simulink model "PVArray_MPPT"  (R2020b)
settings: Solver=VariableStepAuto  StartTime=0.0  StopTime=1  FixedStep=Ts_Power  RelTol=0.001
PreLoadFcn:
  | Ts_Power=5e-4;
  | Slope_Vdc=1;
InitFcn:
  | Ts_Power=50e-6;
  | Tc=1e-5;%break algebraic loop time constant
StopFcn:
  | if exist('I','var') && exist('V','var')
  |    figure(1)
  |    clf
  |    n=find(I>=0);
  |    n=n(end);
  |    Vglobal=V(1:n);
  |    Iglobal=I(1:n);
  | 
  | 
  |    Pglobal=Vglobal.*Iglobal;
  |    n=find(Pglobal==max(Pglobal));
  |    Pmax=Pglobal(n);
  |    Vmp=Vglobal(n);
  |    Imp=Iglobal(n);
  | 
  | 
  |    subplot(211)
  |    plot(Vglobal, Iglobal,Vmp,Imp,'or')
  |    ylabel('Current (A)')
  |    title(sprintf('Global I-V & P-V characteristics\n %s' ,ModuleName))
  | 
  | 
  |    subplot(212)
  |    plot(Vglobal, Pglobal,Vmp,Pmax,'or')
  |    ylabel('Power (W)')
  |    xlabel('Voltage (V)')
  | end
model workspace (MAT data in the model file):
  slope_Vdc = 3.0848387096
libraries: powerlib x60, re_lib x28, simulink x1
(part 2 of 2)

== system PVArray_MPPT/PV2 ==
  Gate : Inport
  Irr : Inport  Port=2
  1PΩ : Constant  Value=1e15
  Ideal Switch : powerlib/Power Electronics/Ideal Switch  Ron=1e-15  Lon=0  IC=0  Rs=1e15  Cs=inf  Measurements=on
  PV1 : re_lib/Solar/PV Array  Npar=1  Nser=1  PlotType=array @ 25 deg.C & specified irradiances  S_vec="[ 1000  500  100 ]"  Temp_C_vec="[ 45 25  ]"  ModuleName=User-defined  PlotWhenSelected=off  Pm=3.9326  Ncell=1  Voc=0.7712096774  Isc=6.18  Vm=0.6676774194  Im=5.89  beta_Voc_pc=-0.2256195755  alpha_Isc_pc=0.04692556634  beta_Voc=-0.00174  alpha_Isc=0.0029  IL=6.2063  I0=6.3357e-13  nI=1.0041  Rsh=6.9252  Rs=0.0032344  RobustModel=on  RobustCellTemperature=25  BAL=on  Tc=1e-5  Tfilter=5e-5
  Terminator : Terminator
  Terminator1 : Terminator
  Variable Resistor2 : powerlib/Elements/Variable Resistor  Rabsmin=1e-3
      settings: SourceProductBaseCode=PS
  + : PMIOPort  Side=Left
  SW : PMIOPort  Port=2  Side=Right
  - : PMIOPort  Port=3  Side=Right
  wires:
  Gate/1 -> Ideal Switch/1
  Irr/1 -> PV1/1
  1PΩ/1 -> Variable Resistor2/1
  Ideal Switch/1 -> Terminator/1
  PV1/1 -> Terminator1/1
  connections:
  Ideal Switch/RConn1 -- SW/RConn1
  Variable Resistor2/RConn1 -- PV1/RConn2 -- -/RConn1
  +/RConn1 -- Variable Resistor2/LConn1 -- Ideal Switch/LConn1 -- PV1/RConn1

== system PVArray_MPPT/PV20 ==
  Gate : Inport
  Irr : Inport  Port=2
  1PΩ : Constant  Value=1e15
  Ideal Switch : powerlib/Power Electronics/Ideal Switch  Ron=1e-15  Lon=0  IC=0  Rs=1e15  Cs=inf  Measurements=on
  PV1 : re_lib/Solar/PV Array  Npar=1  Nser=1  PlotType=array @ 25 deg.C & specified irradiances  S_vec="[ 1000  500  100 ]"  Temp_C_vec="[ 45 25  ]"  ModuleName=User-defined  PlotWhenSelected=off  Pm=3.9326  Ncell=1  Voc=0.7712096774  Isc=6.18  Vm=0.6676774194  Im=5.89  beta_Voc_pc=-0.2256195755  alpha_Isc_pc=0.04692556634  beta_Voc=-0.00174  alpha_Isc=0.0029  IL=6.2063  I0=6.3357e-13  nI=1.0041  Rsh=6.9252  Rs=0.0032344  RobustModel=on  RobustCellTemperature=25  BAL=on  Tc=1e-5  Tfilter=5e-5
  Terminator : Terminator
  Terminator1 : Terminator
  Variable Resistor2 : powerlib/Elements/Variable Resistor  Rabsmin=1e-3
      settings: SourceProductBaseCode=PS
  + : PMIOPort  Side=Left
  SW : PMIOPort  Port=2  Side=Right
  - : PMIOPort  Port=3  Side=Right
  wires:
  Gate/1 -> Ideal Switch/1
  Irr/1 -> PV1/1
  1PΩ/1 -> Variable Resistor2/1
  Ideal Switch/1 -> Terminator/1
  PV1/1 -> Terminator1/1
  connections:
  Ideal Switch/RConn1 -- SW/RConn1
  Variable Resistor2/RConn1 -- PV1/RConn2 -- -/RConn1
  +/RConn1 -- Variable Resistor2/LConn1 -- Ideal Switch/LConn1 -- PV1/RConn1

== system PVArray_MPPT/PV21 ==
  Gate : Inport
  Irr : Inport  Port=2
  1PΩ : Constant  Value=1e15
  Ideal Switch : powerlib/Power Electronics/Ideal Switch  Ron=1e-15  Lon=0  IC=0  Rs=1e15  Cs=inf  Measurements=on
  PV1 : re_lib/Solar/PV Array  Npar=1  Nser=1  PlotType=array @ 25 deg.C & specified irradiances  S_vec="[ 1000  500  100 ]"  Temp_C_vec="[ 45 25  ]"  ModuleName=User-defined  PlotWhenSelected=off  Pm=3.9326  Ncell=1  Voc=0.7712096774  Isc=6.18  Vm=0.6676774194  Im=5.89  beta_Voc_pc=-0.2256195755  alpha_Isc_pc=0.04692556634  beta_Voc=-0.00174  alpha_Isc=0.0029  IL=6.2063  I0=6.3357e-13  nI=1.0041  Rsh=6.9252  Rs=0.0032344  RobustModel=on  RobustCellTemperature=25  BAL=on  Tc=1e-5  Tfilter=5e-5
  Terminator : Terminator
  Terminator1 : Terminator
  Variable Resistor2 : powerlib/Elements/Variable Resistor  Rabsmin=1e-3
      settings: SourceProductBaseCode=PS
  + : PMIOPort  Side=Left
  SW : PMIOPort  Port=2  Side=Right
  - : PMIOPort  Port=3  Side=Right
  wires:
  Gate/1 -> Ideal Switch/1
  Irr/1 -> PV1/1
  1PΩ/1 -> Variable Resistor2/1
  Ideal Switch/1 -> Terminator/1
  PV1/1 -> Terminator1/1
  connections:
  Ideal Switch/RConn1 -- SW/RConn1
  Variable Resistor2/RConn1 -- PV1/RConn2 -- -/RConn1
  +/RConn1 -- Variable Resistor2/LConn1 -- Ideal Switch/LConn1 -- PV1/RConn1

== system PVArray_MPPT/PV22 ==
  Gate : Inport
  Irr : Inport  Port=2
  1PΩ : Constant  Value=1e15
  Ideal Switch : powerlib/Power Electronics/Ideal Switch  Ron=1e-15  Lon=0  IC=0  Rs=1e15  Cs=inf  Measurements=on
  PV1 : re_lib/Solar/PV Array  Npar=1  Nser=1  PlotType=array @ 25 deg.C & specified irradiances  S_vec="[ 1000  500  100 ]"  Temp_C_vec="[ 45 25  ]"  ModuleName=User-defined  PlotWhenSelected=off  Pm=3.9326  Ncell=1  Voc=0.7712096774  Isc=6.18  Vm=0.6676774194  Im=5.89  beta_Voc_pc=-0.2256195755  alpha_Isc_pc=0.04692556634  beta_Voc=-0.00174  alpha_Isc=0.0029  IL=6.2063  I0=6.3357e-13  nI=1.0041  Rsh=6.9252  Rs=0.0032344  RobustModel=on  RobustCellTemperature=25  BAL=on  Tc=1e-5  Tfilter=5e-5
  Terminator : Terminator
  Terminator1 : Terminator
  Variable Resistor2 : powerlib/Elements/Variable Resistor  Rabsmin=1e-3
      settings: SourceProductBaseCode=PS
  + : PMIOPort  Side=Left
  SW : PMIOPort  Port=2  Side=Right
  - : PMIOPort  Port=3  Side=Right
  wires:
  Gate/1 -> Ideal Switch/1
  Irr/1 -> PV1/1
  1PΩ/1 -> Variable Resistor2/1
  Ideal Switch/1 -> Terminator/1
  PV1/1 -> Terminator1/1
  connections:
  Ideal Switch/RConn1 -- SW/RConn1
  Variable Resistor2/RConn1 -- PV1/RConn2 -- -/RConn1
  +/RConn1 -- Variable Resistor2/LConn1 -- Ideal Switch/LConn1 -- PV1/RConn1

== system PVArray_MPPT/PV23 ==
  Gate : Inport
  Irr : Inport  Port=2
  1PΩ : Constant  Value=1e15
  Ideal Switch : powerlib/Power Electronics/Ideal Switch  Ron=1e-15  Lon=0  IC=0  Rs=1e15  Cs=inf  Measurements=on
  PV1 : re_lib/Solar/PV Array  Npar=1  Nser=1  PlotType=array @ 25 deg.C & specified irradiances  S_vec="[ 1000  500  100 ]"  Temp_C_vec="[ 45 25  ]"  ModuleName=User-defined  PlotWhenSelected=off  Pm=3.9326  Ncell=1  Voc=0.7712096774  Isc=6.18  Vm=0.6676774194  Im=5.89  beta_Voc_pc=-0.2256195755  alpha_Isc_pc=0.04692556634  beta_Voc=-0.00174  alpha_Isc=0.0029  IL=6.2063  I0=6.3357e-13  nI=1.0041  Rsh=6.9252  Rs=0.0032344  RobustModel=on  RobustCellTemperature=25  BAL=on  Tc=1e-5  Tfilter=5e-5
  Terminator : Terminator
  Terminator1 : Terminator
  Variable Resistor2 : powerlib/Elements/Variable Resistor  Rabsmin=1e-3
      settings: SourceProductBaseCode=PS
  + : PMIOPort  Side=Left
  SW : PMIOPort  Port=2  Side=Right
  - : PMIOPort  Port=3  Side=Right
  wires:
  Gate/1 -> Ideal Switch/1
  Irr/1 -> PV1/1
  1PΩ/1 -> Variable Resistor2/1
  Ideal Switch/1 -> Terminator/1
  PV1/1 -> Terminator1/1
  connections:
  Ideal Switch/RConn1 -- SW/RConn1
  Variable Resistor2/RConn1 -- PV1/RConn2 -- -/RConn1
  +/RConn1 -- Variable Resistor2/LConn1 -- Ideal Switch/LConn1 -- PV1/RConn1

== system PVArray_MPPT/PV24 ==
  Gate : Inport
  Irr : Inport  Port=2
  1PΩ : Constant  Value=1e15
  Ideal Switch : powerlib/Power Electronics/Ideal Switch  Ron=1e-15  Lon=0  IC=0  Rs=1e15  Cs=inf  Measurements=on
  PV1 : re_lib/Solar/PV Array  Npar=1  Nser=1  PlotType=array @ 25 deg.C & specified irradiances  S_vec="[ 1000  500  100 ]"  Temp_C_vec="[ 45 25  ]"  ModuleName=User-defined  PlotWhenSelected=off  Pm=3.9326  Ncell=1  Voc=0.7712096774  Isc=6.18  Vm=0.6676774194  Im=5.89  beta_Voc_pc=-0.2256195755  alpha_Isc_pc=0.04692556634  beta_Voc=-0.00174  alpha_Isc=0.0029  IL=6.2063  I0=6.3357e-13  nI=1.0041  Rsh=6.9252  Rs=0.0032344  RobustModel=on  RobustCellTemperature=25  BAL=on  Tc=1e-5  Tfilter=5e-5
  Terminator : Terminator
  Terminator1 : Terminator
  Variable Resistor2 : powerlib/Elements/Variable Resistor  Rabsmin=1e-3
      settings: SourceProductBaseCode=PS
  + : PMIOPort  Side=Left
  SW : PMIOPort  Port=2  Side=Right
  - : PMIOPort  Port=3  Side=Right
  wires:
  Gate/1 -> Ideal Switch/1
  Irr/1 -> PV1/1
  1PΩ/1 -> Variable Resistor2/1
  Ideal Switch/1 -> Terminator/1
  PV1/1 -> Terminator1/1
  connections:
  Ideal Switch/RConn1 -- SW/RConn1
  Variable Resistor2/RConn1 -- PV1/RConn2 -- -/RConn1
  +/RConn1 -- Variable Resistor2/LConn1 -- Ideal Switch/LConn1 -- PV1/RConn1

== system PVArray_MPPT/PV25 ==
  Gate : Inport
  Irr : Inport  Port=2
  1PΩ : Constant  Value=1e15
  Ideal Switch : powerlib/Power Electronics/Ideal Switch  Ron=1e-15  Lon=0  IC=0  Rs=1e15  Cs=inf  Measurements=on
  PV1 : re_lib/Solar/PV Array  Npar=1  Nser=1  PlotType=array @ 25 deg.C & specified irradiances  S_vec="[ 1000  500  100 ]"  Temp_C_vec="[ 45 25  ]"  ModuleName=User-defined  PlotWhenSelected=off  Pm=3.9326  Ncell=1  Voc=0.7712096774  Isc=6.18  Vm=0.6676774194  Im=5.89  beta_Voc_pc=-0.2256195755  alpha_Isc_pc=0.04692556634  beta_Voc=-0.00174  alpha_Isc=0.0029  IL=6.2063  I0=6.3357e-13  nI=1.0041  Rsh=6.9252  Rs=0.0032344  RobustModel=on  RobustCellTemperature=25  BAL=on  Tc=1e-5  Tfilter=5e-5
  Terminator : Terminator
  Terminator1 : Terminator
  Variable Resistor2 : powerlib/Elements/Variable Resistor  Rabsmin=1e-3
      settings: SourceProductBaseCode=PS
  + : PMIOPort  Side=Left
  SW : PMIOPort  Port=2  Side=Right
  - : PMIOPort  Port=3  Side=Right
  wires:
  Gate/1 -> Ideal Switch/1
  Irr/1 -> PV1/1
  1PΩ/1 -> Variable Resistor2/1
  Ideal Switch/1 -> Terminator/1
  PV1/1 -> Terminator1/1
  connections:
  Ideal Switch/RConn1 -- SW/RConn1
  Variable Resistor2/RConn1 -- PV1/RConn2 -- -/RConn1
  +/RConn1 -- Variable Resistor2/LConn1 -- Ideal Switch/LConn1 -- PV1/RConn1

== system PVArray_MPPT/PV26 ==
  Gate : Inport
  Irr : Inport  Port=2
  1PΩ : Constant  Value=1e15
  Ideal Switch : powerlib/Power Electronics/Ideal Switch  Ron=1e-15  Lon=0  IC=0  Rs=1e15  Cs=inf  Measurements=on
  PV1 : re_lib/Solar/PV Array  Npar=1  Nser=1  PlotType=array @ 25 deg.C & specified irradiances  S_vec="[ 1000  500  100 ]"  Temp_C_vec="[ 45 25  ]"  ModuleName=User-defined  PlotWhenSelected=off  Pm=3.9326  Ncell=1  Voc=0.7712096774  Isc=6.18  Vm=0.6676774194  Im=5.89  beta_Voc_pc=-0.2256195755  alpha_Isc_pc=0.04692556634  beta_Voc=-0.00174  alpha_Isc=0.0029  IL=6.2063  I0=6.3357e-13  nI=1.0041  Rsh=6.9252  Rs=0.0032344  RobustModel=on  RobustCellTemperature=25  BAL=on  Tc=1e-5  Tfilter=5e-5
  Terminator : Terminator
  Terminator1 : Terminator
  Variable Resistor2 : powerlib/Elements/Variable Resistor  Rabsmin=1e-3
      settings: SourceProductBaseCode=PS
  + : PMIOPort  Side=Left
  SW : PMIOPort  Port=2  Side=Right
  - : PMIOPort  Port=3  Side=Right
  wires:
  Gate/1 -> Ideal Switch/1
  Irr/1 -> PV1/1
  1PΩ/1 -> Variable Resistor2/1
  Ideal Switch/1 -> Terminator/1
  PV1/1 -> Terminator1/1
  connections:
  Ideal Switch/RConn1 -- SW/RConn1
  Variable Resistor2/RConn1 -- PV1/RConn2 -- -/RConn1
  +/RConn1 -- Variable Resistor2/LConn1 -- Ideal Switch/LConn1 -- PV1/RConn1

== system PVArray_MPPT/PV27 ==
  Gate : Inport
  Irr : Inport  Port=2
  1PΩ : Constant  Value=1e15
  Ideal Switch : powerlib/Power Electronics/Ideal Switch  Ron=1e-15  Lon=0  IC=0  Rs=1e15  Cs=inf  Measurements=on
  PV1 : re_lib/Solar/PV Array  Npar=1  Nser=1  PlotType=array @ 25 deg.C & specified irradiances  S_vec="[ 1000  500  100 ]"  Temp_C_vec="[ 45 25  ]"  ModuleName=User-defined  PlotWhenSelected=off  Pm=3.9326  Ncell=1  Voc=0.7712096774  Isc=6.18  Vm=0.6676774194  Im=5.89  beta_Voc_pc=-0.2256195755  alpha_Isc_pc=0.04692556634  beta_Voc=-0.00174  alpha_Isc=0.0029  IL=6.2063  I0=6.3357e-13  nI=1.0041  Rsh=6.9252  Rs=0.0032344  RobustModel=on  RobustCellTemperature=25  BAL=on  Tc=1e-5  Tfilter=5e-5
  Terminator : Terminator
  Terminator1 : Terminator
  Variable Resistor2 : powerlib/Elements/Variable Resistor  Rabsmin=1e-3
      settings: SourceProductBaseCode=PS
  + : PMIOPort  Side=Left
  SW : PMIOPort  Port=2  Side=Right
  - : PMIOPort  Port=3  Side=Right
  wires:
  Gate/1 -> Ideal Switch/1
  Irr/1 -> PV1/1
  1PΩ/1 -> Variable Resistor2/1
  Ideal Switch/1 -> Terminator/1
  PV1/1 -> Terminator1/1
  connections:
  Ideal Switch/RConn1 -- SW/RConn1
  Variable Resistor2/RConn1 -- PV1/RConn2 -- -/RConn1
  +/RConn1 -- Variable Resistor2/LConn1 -- Ideal Switch/LConn1 -- PV1/RConn1

== system PVArray_MPPT/PV28 ==
  Gate : Inport
  Irr : Inport  Port=2
  1PΩ : Constant  Value=1e15
  Ideal Switch : powerlib/Power Electronics/Ideal Switch  Ron=1e-15  Lon=0  IC=0  Rs=1e15  Cs=inf  Measurements=on
  PV1 : re_lib/Solar/PV Array  Npar=1  Nser=1  PlotType=array @ 25 deg.C & specified irradiances  S_vec="[ 1000  500  100 ]"  Temp_C_vec="[ 45 25  ]"  ModuleName=User-defined  PlotWhenSelected=off  Pm=3.9326  Ncell=1  Voc=0.7712096774  Isc=6.18  Vm=0.6676774194  Im=5.89  beta_Voc_pc=-0.2256195755  alpha_Isc_pc=0.04692556634  beta_Voc=-0.00174  alpha_Isc=0.0029  IL=6.2063  I0=6.3357e-13  nI=1.0041  Rsh=6.9252  Rs=0.0032344  RobustModel=on  RobustCellTemperature=25  BAL=on  Tc=1e-5  Tfilter=5e-5
  Terminator : Terminator
  Terminator1 : Terminator
  Variable Resistor2 : powerlib/Elements/Variable Resistor  Rabsmin=1e-3
      settings: SourceProductBaseCode=PS
  + : PMIOPort  Side=Left
  SW : PMIOPort  Port=2  Side=Right
  - : PMIOPort  Port=3  Side=Right
  wires:
  Gate/1 -> Ideal Switch/1
  Irr/1 -> PV1/1
  1PΩ/1 -> Variable Resistor2/1
  Ideal Switch/1 -> Terminator/1
  PV1/1 -> Terminator1/1
  connections:
  Ideal Switch/RConn1 -- SW/RConn1
  Variable Resistor2/RConn1 -- PV1/RConn2 -- -/RConn1
  +/RConn1 -- Variable Resistor2/LConn1 -- Ideal Switch/LConn1 -- PV1/RConn1

== system PVArray_MPPT/PV3 ==
  Gate : Inport
  Irr : Inport  Port=2
  1PΩ : Constant  Value=1e15
  Ideal Switch : powerlib/Power Electronics/Ideal Switch  Ron=1e-15  Lon=0  IC=0  Rs=1e15  Cs=inf  Measurements=on
  PV1 : re_lib/Solar/PV Array  Npar=1  Nser=1  PlotType=array @ 25 deg.C & specified irradiances  S_vec="[ 1000  500  100 ]"  Temp_C_vec="[ 45 25  ]"  ModuleName=User-defined  PlotWhenSelected=off  Pm=3.9326  Ncell=1  Voc=0.7712096774  Isc=6.18  Vm=0.6676774194  Im=5.89  beta_Voc_pc=-0.2256195755  alpha_Isc_pc=0.04692556634  beta_Voc=-0.00174  alpha_Isc=0.0029  IL=6.2063  I0=6.3357e-13  nI=1.0041  Rsh=6.9252  Rs=0.0032344  RobustModel=on  RobustCellTemperature=25  BAL=on  Tc=1e-5  Tfilter=5e-5
  Terminator : Terminator
  Terminator1 : Terminator
  Variable Resistor2 : powerlib/Elements/Variable Resistor  Rabsmin=1e-3
      settings: SourceProductBaseCode=PS
  + : PMIOPort  Side=Left
  SW : PMIOPort  Port=2  Side=Right
  - : PMIOPort  Port=3  Side=Right
  wires:
  Gate/1 -> Ideal Switch/1
  Irr/1 -> PV1/1
  1PΩ/1 -> Variable Resistor2/1
  Ideal Switch/1 -> Terminator/1
  PV1/1 -> Terminator1/1
  connections:
  Ideal Switch/RConn1 -- SW/RConn1
  Variable Resistor2/RConn1 -- PV1/RConn2 -- -/RConn1
  +/RConn1 -- Variable Resistor2/LConn1 -- Ideal Switch/LConn1 -- PV1/RConn1

== system PVArray_MPPT/PV4 ==
  Gate : Inport
  Irr : Inport  Port=2
  1PΩ : Constant  Value=1e15
  Ideal Switch : powerlib/Power Electronics/Ideal Switch  Ron=1e-15  Lon=0  IC=0  Rs=1e15  Cs=inf  Measurements=on
  PV1 : re_lib/Solar/PV Array  Npar=1  Nser=1  PlotType=array @ 25 deg.C & specified irradiances  S_vec="[ 1000  500  100 ]"  Temp_C_vec="[ 45 25  ]"  ModuleName=User-defined  PlotWhenSelected=off  Pm=3.9326  Ncell=1  Voc=0.7712096774  Isc=6.18  Vm=0.6676774194  Im=5.89  beta_Voc_pc=-0.2256195755  alpha_Isc_pc=0.04692556634  beta_Voc=-0.00174  alpha_Isc=0.0029  IL=6.2063  I0=6.3357e-13  nI=1.0041  Rsh=6.9252  Rs=0.0032344  RobustModel=on  RobustCellTemperature=25  BAL=on  Tc=1e-5  Tfilter=5e-5
  Terminator : Terminator
  Terminator1 : Terminator
  Variable Resistor2 : powerlib/Elements/Variable Resistor  Rabsmin=1e-3
      settings: SourceProductBaseCode=PS
  + : PMIOPort  Side=Left
  SW : PMIOPort  Port=2  Side=Right
  - : PMIOPort  Port=3  Side=Right
  wires:
  Gate/1 -> Ideal Switch/1
  Irr/1 -> PV1/1
  1PΩ/1 -> Variable Resistor2/1
  Ideal Switch/1 -> Terminator/1
  PV1/1 -> Terminator1/1
  connections:
  Ideal Switch/RConn1 -- SW/RConn1
  Variable Resistor2/RConn1 -- PV1/RConn2 -- -/RConn1
  +/RConn1 -- Variable Resistor2/LConn1 -- Ideal Switch/LConn1 -- PV1/RConn1

== system PVArray_MPPT/PV5 ==
  Gate : Inport
  Irr : Inport  Port=2
  1PΩ : Constant  Value=1e15
  Ideal Switch : powerlib/Power Electronics/Ideal Switch  Ron=1e-15  Lon=0  IC=0  Rs=1e15  Cs=inf  Measurements=on
  PV1 : re_lib/Solar/PV Array  Npar=1  Nser=1  PlotType=array @ 25 deg.C & specified irradiances  S_vec="[ 1000  500  100 ]"  Temp_C_vec="[ 45 25  ]"  ModuleName=User-defined  PlotWhenSelected=off  Pm=3.9326  Ncell=1  Voc=0.7712096774  Isc=6.18  Vm=0.6676774194  Im=5.89  beta_Voc_pc=-0.2256195755  alpha_Isc_pc=0.04692556634  beta_Voc=-0.00174  alpha_Isc=0.0029  IL=6.2063  I0=6.3357e-13  nI=1.0041  Rsh=6.9252  Rs=0.0032344  RobustModel=on  RobustCellTemperature=25  BAL=on  Tc=1e-5  Tfilter=5e-5
  Terminator : Terminator
  Terminator1 : Terminator
  Variable Resistor2 : powerlib/Elements/Variable Resistor  Rabsmin=1e-3
      settings: SourceProductBaseCode=PS
  + : PMIOPort  Side=Left
  SW : PMIOPort  Port=2  Side=Right
  - : PMIOPort  Port=3  Side=Right
  wires:
  Gate/1 -> Ideal Switch/1
  Irr/1 -> PV1/1
  1PΩ/1 -> Variable Resistor2/1
  Ideal Switch/1 -> Terminator/1
  PV1/1 -> Terminator1/1
  connections:
  Ideal Switch/RConn1 -- SW/RConn1
  Variable Resistor2/RConn1 -- PV1/RConn2 -- -/RConn1
  +/RConn1 -- Variable Resistor2/LConn1 -- Ideal Switch/LConn1 -- PV1/RConn1

== system PVArray_MPPT/PV6 ==
  Gate : Inport
  Irr : Inport  Port=2
  1PΩ : Constant  Value=1e15
  Ideal Switch : powerlib/Power Electronics/Ideal Switch  Ron=1e-15  Lon=0  IC=0  Rs=1e15  Cs=inf  Measurements=on
  PV1 : re_lib/Solar/PV Array  Npar=1  Nser=1  PlotType=array @ 25 deg.C & specified irradiances  S_vec="[ 1000  500  100 ]"  Temp_C_vec="[ 45 25  ]"  ModuleName=User-defined  PlotWhenSelected=off  Pm=3.9326  Ncell=1  Voc=0.7712096774  Isc=6.18  Vm=0.6676774194  Im=5.89  beta_Voc_pc=-0.2256195755  alpha_Isc_pc=0.04692556634  beta_Voc=-0.00174  alpha_Isc=0.0029  IL=6.2063  I0=6.3357e-13  nI=1.0041  Rsh=6.9252  Rs=0.0032344  RobustModel=on  RobustCellTemperature=25  BAL=on  Tc=1e-5  Tfilter=5e-5
  Terminator : Terminator
  Terminator1 : Terminator
  Variable Resistor2 : powerlib/Elements/Variable Resistor  Rabsmin=1e-3
      settings: SourceProductBaseCode=PS
  + : PMIOPort  Side=Left
  SW : PMIOPort  Port=2  Side=Right
  - : PMIOPort  Port=3  Side=Right
  wires:
  Gate/1 -> Ideal Switch/1
  Irr/1 -> PV1/1
  1PΩ/1 -> Variable Resistor2/1
  Ideal Switch/1 -> Terminator/1
  PV1/1 -> Terminator1/1
  connections:
  Ideal Switch/RConn1 -- SW/RConn1
  Variable Resistor2/RConn1 -- PV1/RConn2 -- -/RConn1
  +/RConn1 -- Variable Resistor2/LConn1 -- Ideal Switch/LConn1 -- PV1/RConn1

== system PVArray_MPPT/PV7 ==
  Gate : Inport
  Irr : Inport  Port=2
  1PΩ : Constant  Value=1e15
  Ideal Switch : powerlib/Power Electronics/Ideal Switch  Ron=1e-15  Lon=0  IC=0  Rs=1e15  Cs=inf  Measurements=on
  PV1 : re_lib/Solar/PV Array  Npar=1  Nser=1  PlotType=array @ 25 deg.C & specified irradiances  S_vec="[ 1000  500  100 ]"  Temp_C_vec="[ 45 25  ]"  ModuleName=User-defined  PlotWhenSelected=off  Pm=3.9326  Ncell=1  Voc=0.7712096774  Isc=6.18  Vm=0.6676774194  Im=5.89  beta_Voc_pc=-0.2256195755  alpha_Isc_pc=0.04692556634  beta_Voc=-0.00174  alpha_Isc=0.0029  IL=6.2063  I0=6.3357e-13  nI=1.0041  Rsh=6.9252  Rs=0.0032344  RobustModel=on  RobustCellTemperature=25  BAL=on  Tc=1e-5  Tfilter=5e-5
  Terminator : Terminator
  Terminator1 : Terminator
  Variable Resistor2 : powerlib/Elements/Variable Resistor  Rabsmin=1e-3
      settings: SourceProductBaseCode=PS
  + : PMIOPort  Side=Left
  SW : PMIOPort  Port=2  Side=Right
  - : PMIOPort  Port=3  Side=Right
  wires:
  Gate/1 -> Ideal Switch/1
  Irr/1 -> PV1/1
  1PΩ/1 -> Variable Resistor2/1
  Ideal Switch/1 -> Terminator/1
  PV1/1 -> Terminator1/1
  connections:
  Ideal Switch/RConn1 -- SW/RConn1
  Variable Resistor2/RConn1 -- PV1/RConn2 -- -/RConn1
  +/RConn1 -- Variable Resistor2/LConn1 -- Ideal Switch/LConn1 -- PV1/RConn1

== system PVArray_MPPT/PV8 ==
  Gate : Inport
  Irr : Inport  Port=2
  1PΩ : Constant  Value=1e15
  Ideal Switch : powerlib/Power Electronics/Ideal Switch  Ron=1e-15  Lon=0  IC=0  Rs=1e15  Cs=inf  Measurements=on
  PV1 : re_lib/Solar/PV Array  Npar=1  Nser=1  PlotType=array @ 25 deg.C & specified irradiances  S_vec="[ 1000  500  100 ]"  Temp_C_vec="[ 45 25  ]"  ModuleName=User-defined  PlotWhenSelected=off  Pm=3.9326  Ncell=1  Voc=0.7712096774  Isc=6.18  Vm=0.6676774194  Im=5.89  beta_Voc_pc=-0.2256195755  alpha_Isc_pc=0.04692556634  beta_Voc=-0.00174  alpha_Isc=0.0029  IL=6.2063  I0=6.3357e-13  nI=1.0041  Rsh=6.9252  Rs=0.0032344  RobustModel=on  RobustCellTemperature=25  BAL=on  Tc=1e-5  Tfilter=5e-5
  Terminator : Terminator
  Terminator1 : Terminator
  Variable Resistor2 : powerlib/Elements/Variable Resistor  Rabsmin=1e-3
      settings: SourceProductBaseCode=PS
  + : PMIOPort  Side=Left
  SW : PMIOPort  Port=2  Side=Right
  - : PMIOPort  Port=3  Side=Right
  wires:
  Gate/1 -> Ideal Switch/1
  Irr/1 -> PV1/1
  1PΩ/1 -> Variable Resistor2/1
  Ideal Switch/1 -> Terminator/1
  PV1/1 -> Terminator1/1
  connections:
  Ideal Switch/RConn1 -- SW/RConn1
  Variable Resistor2/RConn1 -- PV1/RConn2 -- -/RConn1
  +/RConn1 -- Variable Resistor2/LConn1 -- Ideal Switch/LConn1 -- PV1/RConn1

== system PVArray_MPPT/PV9 ==
  Gate : Inport
  Irr : Inport  Port=2
  1PΩ : Constant  Value=1e15
  Ideal Switch : powerlib/Power Electronics/Ideal Switch  Ron=1e-15  Lon=0  IC=0  Rs=1e15  Cs=inf  Measurements=on
  PV1 : re_lib/Solar/PV Array  Npar=1  Nser=1  PlotType=array @ 25 deg.C & specified irradiances  S_vec="[ 1000  500  100 ]"  Temp_C_vec="[ 45 25  ]"  ModuleName=User-defined  PlotWhenSelected=off  Pm=3.9326  Ncell=1  Voc=0.7712096774  Isc=6.18  Vm=0.6676774194  Im=5.89  beta_Voc_pc=-0.2256195755  alpha_Isc_pc=0.04692556634  beta_Voc=-0.00174  alpha_Isc=0.0029  IL=6.2063  I0=6.3357e-13  nI=1.0041  Rsh=6.9252  Rs=0.0032344  RobustModel=on  RobustCellTemperature=25  BAL=on  Tc=1e-5  Tfilter=5e-5
  Terminator : Terminator
  Terminator1 : Terminator
  Variable Resistor2 : powerlib/Elements/Variable Resistor  Rabsmin=1e-3
      settings: SourceProductBaseCode=PS
  + : PMIOPort  Side=Left
  SW : PMIOPort  Port=2  Side=Right
  - : PMIOPort  Port=3  Side=Right
  wires:
  Gate/1 -> Ideal Switch/1
  Irr/1 -> PV1/1
  1PΩ/1 -> Variable Resistor2/1
  Ideal Switch/1 -> Terminator/1
  PV1/1 -> Terminator1/1
  connections:
  Ideal Switch/RConn1 -- SW/RConn1
  Variable Resistor2/RConn1 -- PV1/RConn2 -- -/RConn1
  +/RConn1 -- Variable Resistor2/LConn1 -- Ideal Switch/LConn1 -- PV1/RConn1

== system PVArray_MPPT/Variable DC Source ==
  Controlled Voltage Source : powerlib/Electrical Sources/Controlled Voltage Source  Initialize=on  Source_Type=DC  Amplitude=0  Phase=0  Frequency=0  Measurements=None
  Slope Vdc : simulink/Sources/Ramp  slope=Slope_Vdc  start=0  InitialOutput=0
  + : PMIOPort  Side=Left
  - : PMIOPort  Port=2  Side=Left
  wires:
  Slope Vdc/1 -> Controlled Voltage Source/1
  connections:
  Controlled Voltage Source/LConn1 -- -/RConn1
  +/RConn1 -- Controlled Voltage Source/RConn1
